simulink model "Experiment_1_cs_old"  (R2022b)
settings: Solver=ode5  StartTime=0.0  StopTime=30  FixedStep=1/20  RelTol=1e-3
PreLoadFcn:
  | mbxruntime.callbacks.PreLoadFcn(bdroot);
PostLoadFcn:
  | mbxruntime.callbacks.PostLoadFcn(bdroot);
InitFcn:
  | mbxruntime.callbacks.InitFcn(bdroot);
StartFcn:
  | mbxruntime.callbacks.StartFcn(bdroot);
StopFcn:
  | mbxruntime.callbacks.StopFcn(bdroot);
model workspace (MAT data in the model file):
  mbox_table : object (value not decoded)
  model_closed = 0
  sim_status = 0
undefined symbols (not defined in the file or in its folder): blockPath, DiscIntNeverNeededParam, warningInitialVelocity, x0
libraries: PreScanSimulinkLibrary x32, simulink x23, simulink_extras x10
(part 8 of 8)

== matlab function Experiment_1_cs_old/Audi_A8_Sedan_1/perception module/MATLAB Function1 ==
  data: host_x input; obs_x_set_vcs output; host_y input; host_heading_xy input; obs_range input; obs_theta input; obs_velocity input; obs_velocity_heading input; obs_ID input; obs_y_set_vcs output; obs_velocity_set_vcs output; obs_heading_set_vcs output; obs_ID_set output
function [obs_x_set_vcs, obs_y_set_vcs, obs_velocity_set_vcs, obs_heading_set_vcs, obs_ID_set] = ...
    fcn(host_x, host_y, host_heading_xy, obs_range, obs_theta, obs_velocity, obs_velocity_heading, obs_ID)
% 障碍物 VCS 输出 + 遮挡过滤

% =====================
% 初始化输出（固定 10×1）
% =====================
obs_x_set_vcs       = nan(10,1);
obs_y_set_vcs       = nan(10,1);
obs_velocity_set_vcs = nan(10,1);
obs_heading_set_vcs = nan(10,1);
obs_ID_set          = nan(10,1);

% =====================
% 输入角度转换
% =====================
theta_transfer = -obs_theta * pi / 180;
heading_transfer = (-obs_velocity_heading + host_heading_xy * ones(10,1)) * pi/180;

% =====================
% 坐标变换（传感器系 → VCS）
% =====================
x_transfer = obs_range .* cos(theta_transfer);
y_transfer = obs_range .* sin(theta_transfer);

% =====================
% 填入 VCS（包含无效点）
% =====================
for i = 1:length(obs_range)
    if obs_range(i) ~= 0
        obs_x_set_vcs(i)       = x_transfer(i);
        obs_y_set_vcs(i)       = y_transfer(i);
        obs_heading_set_vcs(i) = heading_transfer(i);
        obs_velocity_set_vcs(i)= obs_velocity(i);
        obs_ID_set(i)          = obs_ID(i);
    end
end

% =====================
% ===== 遮挡过滤 =====
% =====================

% 1) 有效点过滤
valid = ~isnan(obs_x_set_vcs);
ox = obs_x_set_vcs(valid);
oy = obs_y_set_vcs(valid);
ov = obs_velocity_set_vcs(valid);
oh = obs_heading_set_vcs(valid);
oid = obs_ID_set(valid);

if isempty(ox)
    return; % 没有障碍物
end

% 2) 计算角度 + 距离
theta = atan2(oy, ox);           % 朝向角 (-pi~pi)
dist  = sqrt(ox.^2 + oy.^2);     % 距离

% 3) 按角度排序（相邻角度判断遮挡）
[theta_sorted, idx] = sort(theta);
ox = ox(idx);
oy = oy(idx);
ov = ov(idx);
oh = oh(idx);
oid = oid(idx);
dist = dist(idx);

% 4) 遮挡过滤（核心）
angle_threshold = deg2rad(5);
coder.extrinsic('disp');
coder.extrinsic('sprintf');

keep = true(size(ox));
for i = 1:length(ox)
    for j = i+1:length(ox)

        if abs(theta_sorted(j) - theta_sorted(i)) > angle_threshold
            break;
        end

        if dist(j) > dist(i)
            keep(j) = false;
            msg = sprintf('Obs %d blocks out Obs %d', oid(i), oid(j));
            disp(msg);
        else
            keep(i) = false;
            msg = sprintf('Obs %d blocks out Obs %d', oid(j), oid(i));
            disp(msg);
        end
    end
end

% 删除被遮挡的障碍物 ★★★★★
ox  = ox(keep);
oy  = oy(keep);
ov  = ov(keep);
oh  = oh(keep);
oid = oid(keep);

% 最终数量
N = length(ox);

% 清空全部槽位
obs_x_set_vcs(:) = nan;
obs_y_set_vcs(:) = nan;
obs_velocity_set_vcs(:) = nan;
obs_heading_set_vcs(:) = nan;
obs_ID_set(:) = nan;

% 回写输出
obs_x_set_vcs(1:N)        = ox;
obs_y_set_vcs(1:N)        = oy;
obs_velocity_set_vcs(1:N) = ov;
obs_heading_set_vcs(1:N)  = oh;
obs_ID_set(1:N)           = oid;

== matlab function Experiment_1_cs_old/Cloud Computing Systerm/PathFollower_Preview_1/LateralController/Calculate delta steering error/eml_delta_steering_error ==
  data: v_x_vehicle input; v_x_vehicle_Min input; t_Preview_LatCtrl input; delta_steeringwheeltotal output; v_y_vehicle input; yawrate_vehicle input; CorneringStiffness_Tyres_Front input; CorneringStiffness_Tyres_Rear input; m_vehicle_total input; inertia_z_vehicle_total input; e_Lat input size=10; Pos_x_CoG_Vehicle input; wheelbase input; RefreshCounter parameter
function delta_steeringwheeltotal = eml_delta_steering_error(v_x_vehicle,v_x_vehicle_Min,t_Preview_LatCtrl,v_y_vehicle,yawrate_vehicle,CorneringStiffness_Tyres_Front,CorneringStiffness_Tyres_Rear,m_vehicle_total,inertia_z_vehicle_total,e_Lat,Pos_x_CoG_Vehicle,wheelbase,RefreshCounter)

delta_steeringwheeltotal = emlfcn_delta_steering_error(v_x_vehicle,v_x_vehicle_Min,t_Preview_LatCtrl,v_y_vehicle,yawrate_vehicle,CorneringStiffness_Tyres_Front,CorneringStiffness_Tyres_Rear,m_vehicle_total,inertia_z_vehicle_total,e_Lat,Pos_x_CoG_Vehicle,wheelbase,RefreshCounter);

% end function
